simulink model "prac4simu"  (R2023a)
settings: Solver=VariableStepAuto  StartTime=0.0  StopTime=10.0  MaxStep=.0001  RelTol=1e-3
values from neighbouring files (symbols this model uses):
  k = 100    [paractica4.m]    (also in parametrosprac_4.m)
  m = 10    [paractica4.m]    (also in parametrosprac_4.m)
settings Model: Creator=User  LastModifiedBy=User

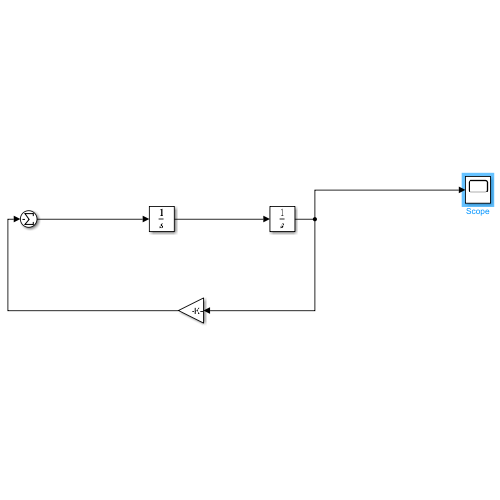
[thumbnail: Simulink's stored preview of the top-level diagram]
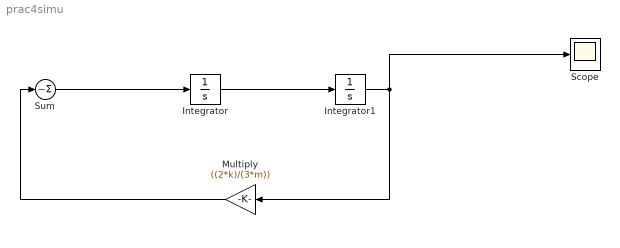
== system prac4simu ==
  Integrator : Integrator  InitialCondition=2
  Integrator1 : Integrator
  Multiply : Gain  Gain=((2*k)/(3*m))
  Scope : Scope
  Sum : Sum  Inputs=-
  wires:
  Sum/1 -> Integrator/1
  Integrator/1 -> Integrator1/1
  Integrator1/1 -> Scope/1, Multiply/1
  Multiply/1 -> Sum/1
